simulink model "GNC_exp"  (R2018a)
settings: Solver=FixedStepAuto  StartTime=0.0  StopTime=50  FixedStep=0.05  MaxStep=0.5  MinStep=0.3  RelTol=10  AbsTol=10
values from neighbouring files (symbols this model uses):
  flightplan = [0,2*dist,height,deg2rad(180) ... (first row only)    [initialize_exp.m]    (also in initialize_race_flighttest.m; initialize_race_realtime.m = [dist,0,height,deg2rad(090))
  g = 9.81    [initialize_exp.m]    (also in initialize_race_flighttest.m; initialize_race_realtime.m)
  max_rot_Z = max_vel*(60)*pi/180    (= 0.523598775598)    [initialize_exp.m]    (also in initialize_race_flighttest.m; initialize_race_realtime.m = 1.57079632679)
  max_theta_X = 75*pi/180    (= 1.308996939)    [initialize_exp.m]    (also in initialize_race_flighttest.m; initialize_race_realtime.m)
  max_theta_Y = 75*pi/180    (= 1.308996939)    [initialize_exp.m]    (also in initialize_race_flighttest.m; initialize_race_realtime.m)
  max_v_Z = 2*max_vel    (= 1)    [initialize_exp.m]    (also in initialize_race_flighttest.m; initialize_race_realtime.m = 3)
  max_vel = 0.5    [initialize_exp.m]    (also in initialize_race_flighttest.m; initialize_race_realtime.m = 1.5)
  spline_init = [P0;P1;P2;P3]    [initialize_exp.m]    (also in initialize_race_flighttest.m; initialize_race_realtime.m)
undefined symbols (not defined in the file or in its folder): eul, HFOV, pos, two_std_dev_init, two_std_dev_thres, vel, VFOV, WP_list_init
libraries: sharedtransform x3, aerolibutil x2, simulink x1
(part 2 of 2)

== system GNC_exp/Navigation/calculate desired/calculate direction B'(d)/Make Unit ==
  Vector : Inport
  Multiply : Product
  Reciprocal Sqrt : Sqrt  Operator=rSqrt  SaturateOnIntegerOverflow=on
  Square : Math  Operator=square  SaturateOnIntegerOverflow=on
  Sum of Elements : Sum  Inputs=+
  Transpose : Math  Operator=transpose  SaturateOnIntegerOverflow=on
  Unit Vector : Outport
  wires:
  Reciprocal Sqrt/1 -> Multiply/1
  Vector/1 -> Square/1, Multiply/2
  Square/1 -> Sum of Elements/1
  Multiply/1 -> Transpose/1
  Sum of Elements/1 -> Reciprocal Sqrt/1
  Transpose/1 -> Unit Vector/1

== system GNC_exp/Navigation/calculate desired/calculate direction B'(d)/old, quadratic ==
  note: B'(d) = 2(1-d)(P1-P0) + 2d(P2-P1) = 2*(dP0-2dP1+dP2+P1-P0)
  d : Inport
  P0 : Inport  Port=2
  P1 : Inport  Port=3
  P2 : Inport  Port=4
  vel : Inport  Port=5
  Add1 : Sum  Commented=on  Inputs=+--++-
  Atan1 : Trigonometry  Commented=on  Operator=atan2
  Constant1 : Constant  Commented=on  Value=0
  Constant2 : Constant  Commented=on  Value=0
  Matrix Multiply : Product  Commented=on  Inputs=/*  Multiplication=Matrix(*)
  Product : Product  Commented=on
  Product1 : Product  Commented=on
  Product2 : Product  Commented=on
  Rotation Angles to Direction Cosine Matrix1 : sharedtransform/Rotation Angles to Direction Cosine Matrix  Commented=on  rotationOrder=ZYX  aMode=aMode
      settings: SourceProductBaseCode=AE
  Selector7 : Selector  Commented=on  IndexMode=Zero-based  InputPortWidth=3  IndexOptions=Index vector (dialog)  Indices=1  OutputSizes=1
  Selector8 : Selector  Commented=on  IndexMode=Zero-based  InputPortWidth=3  IndexOptions=Index vector (dialog)  Indices=0  OutputSizes=1
  Vector Concatenate : Concatenate  Commented=on  NumInputs=3
  Vector Concatenate1 : Concatenate  Commented=on  NumInputs=3
  Out1 : Outport
  wires:
  Product2/1 -> Add1/4
  P1/1 -> Add1/5, Product1/2
  Rotation Angles to Direction Cosine Matrix1/1 -> Matrix Multiply/1  "rot matrix"
  P2/1 -> Product2/2
  Add1/1 -> Selector8/1, Selector7/1
  Product/1 -> Add1/1
  P0/1 -> Add1/6, Product/2
  d/1 -> Product2/1, Product1/1, Product/1
  Constant1/1 -> Vector Concatenate/2, Vector Concatenate/3
  Vector Concatenate1/1 -> Matrix Multiply/2
  Product1/1 -> Add1/3, Add1/2
  Vector Concatenate/1 -> Rotation Angles to Direction Cosine Matrix1/1
  Selector7/1 -> Atan1/1
  vel/1 -> Vector Concatenate1/1
  Constant2/1 -> Vector Concatenate1/2, Vector Concatenate1/3
  Matrix Multiply/1 -> Out1/1
  Selector8/1 -> Atan1/2
  Atan1/1 -> Vector Concatenate/1  "yaw"

== system GNC_exp/Navigation/calc v/Create Path Frame/Make X Vector/Make Unit ==
  Vector : Inport
  Multiply : Product
  Reciprocal Sqrt : Sqrt  Operator=rSqrt  SaturateOnIntegerOverflow=on
  Square : Math  Operator=square  SaturateOnIntegerOverflow=on
  Sum of Elements : Sum  Inputs=+
  Unit Vector : Outport
  wires:
  Reciprocal Sqrt/1 -> Multiply/1
  Vector/1 -> Square/1, Multiply/2
  Square/1 -> Sum of Elements/1
  Multiply/1 -> Unit Vector/1
  Sum of Elements/1 -> Reciprocal Sqrt/1

== system GNC_exp/Navigation/calc v/Create Path Frame/Make Y Vector/Make Unit ==
  Vector : Inport
  Multiply : Product
  Reciprocal Sqrt : Sqrt  Operator=rSqrt  SaturateOnIntegerOverflow=on
  Square : Math  Operator=square  SaturateOnIntegerOverflow=on
  Sum of Elements : Sum  Inputs=+
  Unit Vector : Outport
  wires:
  Reciprocal Sqrt/1 -> Multiply/1
  Vector/1 -> Square/1, Multiply/2
  Square/1 -> Sum of Elements/1
  Multiply/1 -> Unit Vector/1
  Sum of Elements/1 -> Reciprocal Sqrt/1

== system GNC_exp/Navigation/calc v/Create Path Frame/Make Z Vector/Make Unit ==
  Vector : Inport
  Multiply : Product
  Reciprocal Sqrt : Sqrt  Operator=rSqrt  SaturateOnIntegerOverflow=on
  Square : Math  Operator=square  SaturateOnIntegerOverflow=on
  Sum of Elements : Sum  Inputs=+
  Unit Vector : Outport
  wires:
  Reciprocal Sqrt/1 -> Multiply/1
  Vector/1 -> Square/1, Multiply/2
  Square/1 -> Sum of Elements/1
  Multiply/1 -> Unit Vector/1
  Sum of Elements/1 -> Reciprocal Sqrt/1

== matlab function GNC_exp/Guidance/filter_WP_moving_av1 ==
  data: WP_list_out output; WP_idx_out output; WP_list_in input; WP_idx_in input; WP_std_dev_in input; dist_old_raw input; WP_current_pos input; WP_current_eul input; WP_std_dev_out output; init_std_dev input; flightplan input
function [WP_list_out, WP_idx_out, WP_std_dev_out] = filter_WP(WP_list_in, WP_idx_in, WP_std_dev_in, dist_old_raw, WP_current_pos, WP_current_eul, init_std_dev, flightplan)
    
%     WP_list_out = zeros(4,4);
%     WP_std_dev_out = zeros(4,1);
   
    % catch state transition
    WP_idx_out = WP_idx_in;
    if dist_old_raw > 1
        disp('new state')
        WP_idx_out = WP_idx_out+1;
        if WP_idx_out == size(WP_list_in,1)
            WP_idx_out = 0;
        end
        WP_std_dev_in = init_std_dev;
    end
    
    WP_std_dev_out = WP_std_dev_in;
    
    % check if there is gate information
    if isequal(WP_current_eul, zeros(1,3)) || isequal(WP_current_eul, zeros(3,1))
        % no gate info
%         disp('gate_global - no corners')
        WP_list_out = WP_list_in;
    else
        % gate info, update WP
%         disp('gate_global - update')
%         WP_current_ori
        lambda = 0.1;
        
        WP_average = WP_list_in(WP_idx_out+1,:)';
        WP_current = [WP_current_pos; WP_current_eul(1)];
       
        delta = WP_current-WP_average;
        delta(4) = angle_add(WP_current(4),-WP_average(4));
        if delta(4) > pi/2
            delta(4) = delta(4)-pi;
        elseif delta(4) < -pi/2
            delta(4) = delta(4)+pi;
        end
        std = abs(delta) ./ (WP_std_dev_out); 
    
        alpha = lambda.^(std);
        alpha = min(alpha, lambda);
%         alpha = max(alpha, 0.001);
        WP_average(1:3) = WP_average(1:3) + alpha(1:3).*delta(1:3);
        WP_average(4) = angle_add(WP_average(4),alpha(4)*delta(4));
        
        WP_std_dev_out = sqrt((1-alpha).*(WP_std_dev_out.^2+alpha.*delta.*delta));

        %WP_list_out(WP_idx_out+1,:) = WP_average;
        
        % update all WP based on new estimate
        WP_list_out = WP_list_in;
        WP_list_out(WP_idx_out+1,:) = WP_average;
        for i = WP_idx_out+2:size(WP_list_in,1)
            WP_list_out(i,1:3) = WP_list_out(i-1,1:3) + flightplan(i,1:3);
            WP_list_out(i,4) = flightplan(i,4);
        end
        if WP_idx_out ~= 0
            WP_list_out(1,1:3) = WP_list_out(end,1:3) + flightplan(1,1:3);
            WP_list_out(1,4) = flightplan(1,4);
            for i = 2:WP_idx_out
                WP_list_out(i,1:3) = WP_list_out(i-1,1:3) + flightplan(i,1:3);
                WP_list_out(i,4) = flightplan(i,4);
            end
        end
        
    end
end

function sum = angle_add(a1,a2)
    sum = atan2(sin(a1+a2),cos(a1+a2));
end



% 
%         if norm(WP_current_pos' - WP_average_pos) < 0.7
%             WP_average_pos = alpha*WP_current_pos' + (1-alpha)*WP_average_pos;
%             WP_current_hdg = WP_current_ori(1);
%             WP_average_hdg = atan2(alpha*sin(WP_current_hdg) + (1-alpha)*sin(WP_average_hdg), ...
%                 alpha*cos(WP_current_hdg) + (1-alpha)*cos(WP_average_hdg));
%             WP_average = [WP_average_pos, WP_average_hdg];
%             WP_list_out(state0_out+1,:) = WP_average;
%         end

== matlab function GNC_exp/Initialize/reset_plot ==
function reset_plot()
coder.extrinsic('quiver3')
coder.extrinsic('legend')
close all;
figure('units','normalized','outerposition',[0 0 0.5 1])
hold on
grid on
axis equal

legends=zeros(12,1);
legends(1)=plot3(0,0,-100,'m.','MarkerSize',7);
legends(2)=plot3(0,0,-100,'k.','MarkerSize',5);
legends(3)=quiver3(0,0,-100,0,0,0,0,'c','MaxHeadSize',1,'LineWidth',2);
legends(4)=quiver3(0,0,-100,0,0,0,0,'r','MaxHeadSize',1,'LineWidth',2);
legends(5)=plot3(0,0,-100,':','Color',[1,0.7,0],'LineWidth',2);
legends(6)=plot3(0,0,-100,'kx-','LineWidth',1.2,'MarkerIndices',1,'MarkerSize',10);
legends(7)=plot3(0,0,-100,'r--','LineWidth',1.5);
legends(8)=plot3(0,0,-100,'g--','LineWidth',1.5);
legends(9)=plot3(0,0,-100,'b--','LineWidth',1.5);
legends(10)=plot3(0,0,-100,'b+-','LineWidth',1.2,'MarkerIndices',1,'MarkerSize',10);
legends(11)=quiver3(0,0,-100,0,0,0,0,'b','MaxHeadSize',1,'LineWidth',2);
legends(12)=plot3(0,0,-100,':r','LineWidth',1);
legend(legends(1:12),'flown track','ground track','inactive WP +ori','active WP +ori','spline','drone pos+vel','drone x','drone y','drone z','des pos+vel','measured WP','std dev (x,y,th)','Location','eastoutside','AutoUpdate','off')

for i=1:25
    plot3(0,0,-100,'.')
end

% axis([-5,5,-5,5,-2,2])
axis([-2,6,-3,1,-1,3])
% axis([1,4,-2,2,0,4])
%view(-20,40) % 3D view
view(-90,90) % top view
%view(-90,0) % front view
xlabel('x')
ylabel('y')
zlabel('z')

== matlab function GNC_exp/Navigation/select d ==
  data: d_old input; d_old output; std_dev input; two_std_dev_thres input
function d_old = select_d(d_old, std_dev, two_std_dev_thres)

two_std_dev_max = 2*max(std_dev.*[1;1;1;1/(40*pi/180)]);

if two_std_dev_max > two_std_dev_thres
    d_old = 0;
end

== matlab function GNC_exp/Plot ==
  data: inbus input
function plot3d(inbus)
%#codegen
coder.extrinsic('delete')
% coder.extrinsic('ellipsoid')
% coder.extrinsic('viscircles')
% coder.extrinsic('quiver3')
% coder.extrinsic('legend')

drone_vel = inbus.state.vel;
drone_pos = inbus.state.pos;
drone_ori = inbus.state.eul;
WP_curr_eul = inbus.WP_curr.eul;
WP_curr_pos = inbus.WP_curr.pos;
SP_des_vel = inbus.SP_des.vel;
SP_des_pos = inbus.SP_des.pos;
WP_idx = inbus.WP_all.idx + 1;
WP_list = inbus.WP_all.list;
effort = inbus.effort;
std_dev = inbus.std_dev;
current_spline = inbus.current_spline;

children = get(gca, 'children');
amount = 12+size(WP_list,1);
delete(children(1:amount));

P0 = current_spline(1,:);
P1 = current_spline(2,:);
P2 = current_spline(3,:);
P3 = current_spline(4,:);

% flown track + ground track
plot3(drone_pos(1),drone_pos(2),drone_pos(3),'m.','MarkerSize',7); %1
% plot3(drone_pos(1),drone_pos(2),0,'k.','MarkerSize',5); %2

% all WPts + ori
% quiver3 (WP_list(:,1),WP_list(:,2),WP_list(:,3),cos(WP_list(:,4)),sin(WP_list(:,4)),zeros(4,1),0,'c','MaxHeadSize',1,'LineWidth',2); %3
for i = 1:size(WP_list,1)
    if i == WP_idx
        continue
    end
    plot3(WP_list(i,1)+[0 cos(WP_list(i,4))],WP_list(i,2)+[0 sin(WP_list(i,4))],WP_list(i,3)+[0 0],'c+-','LineWidth',2,'MarkerIndices',2); %3
end

% WP average pos+ori
% quiver3(P2(1),P2(2),P2(3),cos(P2(4)),sin(P2(4)),0,0,'r','MaxHeadSize',1,'LineWidth',2); %4
plot3(WP_list(WP_idx,1)+[0 cos(WP_list(WP_idx,4))],WP_list(WP_idx,2)+[0 sin(WP_list(WP_idx,4))],WP_list(WP_idx,3)+[0 0],'r+-','LineWidth',2,'MarkerIndices',2); %3

% spline
d = (0:0.05:1)';
% u = ones(1,3);
% spline_pos_quad = (1-d)*u.*((1-d)*P0+d*P1)+d*u.*((1-d)*P1 + d*P2);
spline_pos_cubic = (1-d).^3*P0 + 3*(1-d).^2.*d*P1 + 3*(1-d).*d.^2*P2 + d.^3*P3;
plot3(spline_pos_cubic(:,1),spline_pos_cubic(:,2),spline_pos_cubic(:,3),':','Color',[1,0.7,0],'LineWidth',2); %5
plot3(current_spline(:,1),current_spline(:,2),current_spline(:,3),'og')

% drone pos+vel
plot3(drone_pos(1)+[0 drone_vel(1)],drone_pos(2)+[0 drone_vel(2)],drone_pos(3)+[0 drone_vel(3)],'kx-','LineWidth',1.2,'MarkerIndices',1,'MarkerSize',10); %6

% drone ori
gRb = eul2rotm([drone_ori(3),drone_ori(2),drone_ori(1)]);
length = 1;
x_bebop = gRb*[length;0;0];
y_bebop = gRb*[0;length;0];
z_bebop = gRb*[0;0;length];
plot3(drone_pos(1)+x_bebop(1)*[0.2 1],drone_pos(2)+x_bebop(2)*[0.2 1],drone_pos(3)+x_bebop(3)*[0.2 1],'r:','LineWidth',1.5); %7
plot3(drone_pos(1)+y_bebop(1)*[0.2 1],drone_pos(2)+y_bebop(2)*[0.2 1],drone_pos(3)+y_bebop(3)*[0.2 1],'g:','LineWidth',1.5); %8
plot3(drone_pos(1)+z_bebop(1)*[0.2 1],drone_pos(2)+z_bebop(2)*[0.2 1],drone_pos(3)+z_bebop(3)*[0.2 1],'b:','LineWidth',1.5); %9

% nav pt pos+vel, (yaw)
plot3(SP_des_pos(1)+[0 SP_des_vel(1)],SP_des_pos(2)+[0 SP_des_vel(2)],SP_des_pos(3)+[0 SP_des_vel(3)],'b+-','LineWidth',1.2,'MarkerIndices',1,'MarkerSize',10); %10
% plot3(WP_pos(1)+[0 0.5*cos(WP_yaw)],WP_pos(2)+[0 0.5*sin(WP_yaw)],WP_pos(3)+[0 0],'r-','LineWidth',1)

% WP current pos + ori
if isequal(WP_curr_eul, zeros(1,3)) || isequal(WP_curr_eul, zeros(3,1))
    % no gate info
    WP_curr_pos = [0,0,-100]';
    x_gate = WP_curr_eul;
else   
    gate_rot = eul2rotm(WP_curr_eul');
    x_gate = gate_rot(:,1);
end
% quiver3(gate_pos_global(1),gate_pos_global(2),gate_pos_global(3),x_gate(1),x_gate(2),x_gate(3),0,'b','MaxHeadSize',1,'LineWidth',2); %11
plot3(WP_curr_pos(1)+[0 x_gate(1)],WP_curr_pos(2)+[0 x_gate(2)],WP_curr_pos(3)+[0 x_gate(3)],'b+-','LineWidth',2,'MarkerIndices',2); %3

% effort
effort_gl = ones(4,1) * drone_pos' + [zeros(1,3);
    x_bebop'*effort(1);
    y_bebop'*effort(2);
    z_bebop'*effort(3)];
plot3(effort_gl([1 2],1),effort_gl([1 2],2),effort_gl([1 2],3),'r-','LineWidth',2);
plot3(effort_gl([1 3],1),effort_gl([1 3],2),effort_gl([1 3],3),'g-','LineWidth',2);
plot3(effort_gl([1 4],1),effort_gl([1 4],2),effort_gl([1 4],3),'b-','LineWidth',2);

% WP std dev
two_std_dev = 2*std_dev;
r=linspace(WP_list(WP_idx,4),WP_list(WP_idx,4)+2*pi,4*4*2+1)';
angle_std_dev_length=0.6;
angle_std_dev_draw = [WP_list(WP_idx,1:3);
    WP_list(WP_idx,1:3)+angle_std_dev_length*[cos(WP_list(WP_idx,4)+two_std_dev(4)), sin(WP_list(WP_idx,4)+two_std_dev(4)), 0];
    WP_list(WP_idx,1:3);
    WP_list(WP_idx,1:3)+angle_std_dev_length*[cos(WP_list(WP_idx,4)-two_std_dev(4)), sin(WP_list(WP_idx,4)-two_std_dev(4)), 0];
    WP_list(WP_idx,1:3);
    WP_list(WP_idx,1)+two_std_dev(1)*cos(atan2(two_std_dev(1)/two_std_dev(2)*sin(r),cos(r))), WP_list(WP_idx,2)+two_std_dev(2)*sin(atan2(two_std_dev(1)/two_std_dev(2)*sin(r),cos(r))), WP_list(WP_idx,3)+0*r];
d = angle_std_dev_draw;
plot3(d(:,1),d(:,2),d(:,3),':r','LineWidth',1); %12
% [ellx,elly,ellz] = ellipsoid(P2(1),P2(2),P2(3),3*std_dev(1),3*std_dev(2),3*std_dev(3),20);
% surf(ellx,elly,ellz,ellz,'FaceAlpha',0.5)

% legend
% legend(legends(1:12),'flown track','ground track','inactive WP +ori','active WP +ori','spline','drone pos+vel','drone x','drone y','drone z','des pos+vel','measured WP','std dev (x,y,th)','Location','eastoutside')

== matlab function GNC_exp/Guidance/select_WP ==
  data: WP_average output; WP_list input; WP_idx input
function WP_average = select_WP(WP_list, WP_idx)
    WP_average=zeros(1,4);
    WP_last=zeros(1,4);
    
    WP_average = WP_list(WP_idx+1,:);
    if WP_idx > 0
        WP_last = WP_list(WP_idx,:);
    else
        WP_last = WP_list(end,:);
    end
end

== matlab function GNC_exp/Guidance/create_spline ==
  data: old_spline input; WP_average input; current_spline output size=[4,3]; std_dev input; d_old_raw input; two_std_dev_thres input; VFOV input; HFOV input
function current_spline = create_spline(old_spline, WP_average, std_dev, d_old_raw, two_std_dev_thres, VFOV, HFOV)

two_std_dev_hor = 2*max(std_dev(1:2));
two_std_dev_vert = 2*max(std_dev(3));
two_std_dev_hor = min(2,two_std_dev_hor);
two_std_dev_vert = min(2,two_std_dev_vert);
two_std_dev_max = 2*max(std_dev.*[1;1;1;1/(40*pi/180)]);

% d_old = mod(d_old_raw,1);

SP_pos = (1-d_old_raw)^3*old_spline(1,:) + 3*(1-d_old_raw)^2*d_old_raw*old_spline(2,:) + 3*(1-d_old_raw)*d_old_raw^2*old_spline(3,:) + d_old_raw^3*old_spline(4,:);
SP_vel = 3*(1-d_old_raw)^2*(old_spline(2,:)-old_spline(1,:)) + 6*(1-d_old_raw)*d_old_raw*(old_spline(3,:)-old_spline(2,:)) + 3*d_old_raw^2*(old_spline(4,:)-old_spline(3,:));
SP_vel0= old_spline(2,:)-old_spline(1,:);

WP_gate = WP_average;
offsetH = (two_std_dev_hor+0.7)/sin(HFOV/2);
offsetV = (two_std_dev_vert+0.7)/tan(VFOV/2);
offsetMAX = max(offsetH,offsetV);
if two_std_dev_max > two_std_dev_thres
    WP1 = [SP_pos, atan2(SP_vel(2),SP_vel(1))];
    WP2 = WP_gate(1:4);
    WP2(1:3) = WP_gate(1:3) - offsetMAX*[cos(WP2(4)) sin(WP2(4)) 0];
else
    WP1 = [old_spline(1,:), atan2(SP_vel0(2),SP_vel0(1))];
    WP2 = WP_gate(1:4);
end
    

%% position cubic spline start at supposed pos, random values
% % B(d) = (1-d)^3*P0 + 3(1-d)^2*d*P1 + 3(1-d)*d^2*P2 + d^3*P3
% % B'(d) = 3(1-d)^2(P1-P0) + 6*(1-d)*d*(P2-P1) + 3d^2(P3-P2)
% 
% % B(0) = P0
% % B(1) = P3
% 
% P0 = WP1(1:3);
% P3 = WP2(1:3);
% hdg0 = WP1(4);
% hdg3 = WP2(4);
% 
% m = norm(P0-P3)-1;
% m = max(0.01,m);+
% P1 = [P0(1)+m*cos(hdg0), P0(2)+m*sin(hdg0), P3(3)];
% 
% offset2 = (std_dev_factor+0.7)/sin(HFOV/2*0.999);
% P2 = WP_average(1:3) - (offset2+1*(offset2-offset1))*[cos(hdg3) sin(hdg3) 0];
%           
% % n = 3-norm(P0-WP_average(1:3));
% % n = max(0.001,n);
% % P2 = P3 - n*[cos(WP2(4)) sin(WP2(4)) 0];
% 
% current_spline = [P0; P1; P2; P3];

%% cube with m = n
% % B(d) = (1-d)^3*P0 + 3(1-d)^2*d*P1 + 3(1-d)*d^2*P2 + d^3*P3
% % B'(d) = 3(1-d)^2(P1-P0) + 6*(1-d)*d*(P2-P1) + 3d^2(P3-P2)
% 
% % B(0) = P0
% % B(1) = P3
% 
% P0 = WP1(1:3);
% P3 = WP2(1:3);
% hdg0 = WP1(4);
% hdg3 = WP2(4);
% 
% % g1: P0 + m*[cos(hdg0);sin(hdg0);0]
% % g2: P3 - n*[cos(hdg3);sin(hdg3);0]
% 
% % m*f(hdg0)+n*f(hdg3) +P0-P3 = 0
% % m*(f(hdg0)+f(hdg3)) +P0-P3 = 0
% 
% % m*(c0+c3)+P0(1)-P3(1)=0
% % m = (P3(1)-P0(1) )/(cos(hdg0)+cos(hdg3))
% 
% m = (P3(1)-P0(1) )/(cos(hdg0)+cos(hdg3));
% P1 = P0 + [m*cos(hdg0), m*sin(hdg0), 1*(P3(3)-P0(3))];
% P2 = P3 - [m*cos(hdg3), m*sin(hdg3), 0              ];
% 
% current_spline = [P0; P1; P2; P3];

%% cube without m=n
% % B(d) = (1-d)^3*P0 + 3(1-d)^2*d*P1 + 3(1-d)*d^2*P2 + d^3*P3
% % B'(d) = 3(1-d)^2(P1-P0) + 6*(1-d)*d*(P2-P1) + 3d^2(P3-P2)
% 
% % B(0) = P0
% % B(1) = P3
% 
% P0 = WP1(1:3);
% P3 = WP2(1:3);
% hdg0 = WP1(4);
% hdg3 = WP2(4);
% 
% % g1: P0 + m*[cos(hdg0);sin(hdg0);0]
% % g2: P3 - n*[cos(hdg3);sin(hdg3);0]
% 
% % m*cos(hdg0)+n*cos(hdg3) +P0(1)-P3(1) = 0
% % m*sin(hdg0)+n*sin(hdg3) +P0(2)-P3(2) = 0
% 
% A = [cos(hdg0) cos(hdg3);
%      sin(hdg0) sin(hdg3)];
% b = -[P0(1)-P3(1);
%     P0(2)-P3(2)];
% r = A\b;
% m = r(1);
% n = r(2);
% P1 = P0 + [m*cos(hdg0), m*sin(hdg0), 1*(P3(3)-P0(3))];
% P2 = P3 - [n*cos(hdg3), n*sin(hdg3), 0];
% 
% current_spline = [P0; P1; P2; P3];

%% cube, m and n from dist
% B(d) = (1-d)^3*P0 + 3(1-d)^2*d*P1 + 3(1-d)*d^2*P2 + d^3*P3
% B'(d) = 3(1-d)^2(P1-P0) + 6*(1-d)*d*(P2-P1) + 3d^2(P3-P2)

% B(0) = P0
% B(1) = P3

P0 = WP1(1:3);
P3 = WP2(1:3);
hdg0 = WP1(4);
hdg3 = WP2(4);

% dist_fly = norm(P0-P3);
% dist_nofly = norm(WP_gate(1:3)-P3);
% fact_nofly = max(0.25,sqrt(dist_nofly/2));
% 
% m = dist_fly/4*fact_nofly;
% n = dist_fly/4/fact_nofly;

l_F = norm(P0-P3);
l_TW = norm(WP_gate(1:3)-P3);

m = l_F*min(1/10+l_TW/10,1/2);
n = l_F*max(1-l_TW/2,1/10);

P1 = P0 + [m*cos(hdg0), m*sin(hdg0), 1*(P3(3)-P0(3))];
P2 = P3 - [n*cos(hdg3), n*sin(hdg3), 0];

current_spline = [P0; P1; P2; P3];
end

== matlab function GNC_exp/Guidance/filter_WP_moving_av ==
  data: WP_list_out output; WP_idx_out output; WP_list_in input; WP_idx_in input; dist_old_raw input; WP_current_pos input; WP_current_eul input; WP_std_dev_out output; WP_est_out output; WP_P_mat_out output; two_init_std_dev input; WP_list_const input; WP_est_in input; WP_P_mat_in input
function [WP_list_out, WP_idx_out, WP_std_dev_out, WP_est_out, WP_P_mat_out] = ...
    filter_WP(WP_list_in, WP_idx_in, dist_old_raw, WP_current_pos, WP_current_eul, two_init_std_dev, WP_list_const, WP_est_in, WP_P_mat_in)
    
    mean_var = diag(0.2*ones(4,1));
    
    % catch script start
    if isequal(WP_P_mat_in,ones(4,4))
        WP_P_mat_in = diag((two_init_std_dev/2).^2);
        WP_est_in = WP_list_const(1,:)';
    end
    
    % catch state transition
    WP_idx_out = WP_idx_in;
    if dist_old_raw > 1
        disp('new state')
        WP_idx_out = WP_idx_out+1;
        if WP_idx_out == size(WP_list_in,1)
            WP_idx_out = 0;
        end
        WP_est_in = WP_list_const(WP_idx_out+1,:)';
        %WP_current_gate_in = WP_list_const(WP_idx_out+1,:)';
        WP_P_mat_in = diag((two_init_std_dev/2).^2);
    end
    WP_current_gate = WP_list_const(WP_idx_out+1,:)';
    WP_list_out = WP_list_in;
    
    WP_P_mat_out = WP_P_mat_in;
    WP_std_dev_out = sqrt(diag(WP_P_mat_out));
    
    WP_est_out = WP_est_in;
    
   
    if WP_current_eul(1) > WP_current_gate(4) + pi/2
        euler_used = WP_current_eul(1)-pi;
    elseif WP_current_eul(1) < WP_current_gate(4)-pi/2
        euler_used = WP_current_eul(1)+pi;
    else
        euler_used = WP_current_eul(1);
    end
        
    % check if there is gate information
    if isequal(WP_current_eul, zeros(1,3)) || isequal(WP_current_eul, zeros(3,1))
        % no gate info
        %         disp('gate_global - no corners')
        
    else

        
        if (norm(WP_current_pos(1:2) - WP_current_gate(1:2)) > 2.0) ||...
                WP_current_pos(1) - WP_est_in(1) > 3*sqrt(WP_P_mat_in(1,1)) || ...
                WP_current_pos(2) - WP_est_in(2) > 3*sqrt(WP_P_mat_in(2,2))
                %sqrt(WP_P_mat_in(4,4)) < 0.1 && ...
                %sqrt(WP_P_mat_in(3,3)) < 0.1 && ...
                %sqrt(WP_P_mat_in(2,2)) < 0.1 && ...
                %sqrt(WP_P_mat_in(1,1)) < 0.1) || WP_idx_out ~= WP_idx_out
            %WP_current = [WP_current_pos; WP_current_eul(1)];
            
            %K_gain = WP_P_mat_in*inv(WP_P_mat_in + mean_var);
            
            WP_est_out = WP_est_in;% + K_gain*(WP_current - WP_est_in);
            WP_P_mat_out = WP_P_mat_in;
            
            WP_list_out(WP_idx_out+1,:) = WP_est_out';
            WP_std_dev_out = sqrt(diag(WP_P_mat_out));
            
        else
            
            WP_current = [WP_current_pos; euler_used];
            
            K_gain = WP_P_mat_in*inv(WP_P_mat_in + mean_var);
            
            delta = WP_current-WP_est_in;
            delta(4) = WP_current(4)-WP_est_in(4); %angle_add(WP_current(4),-WP_est_in(4));
            
            WP_est_out(1:3) = WP_est_in(1:3) + K_gain(1:3,:)*(delta);
            WP_est_out(4) = WP_est_in(4) + K_gain(4,:)*delta; %angle_add(WP_est_in(4),K_gain(4,:)*delta);
            WP_P_mat_out = (eye(4) - K_gain)*WP_P_mat_in;
            
            WP_list_out(WP_idx_out+1,:) = WP_est_out';
            WP_std_dev_out = sqrt(diag(WP_P_mat_out));
        end

%         lambda = 0.1;
%         
%         WP_average = WP_list_out(WP_idx_out+1,:)';
%         
%        
%         delta = WP_current-WP_average;
%         delta(4) = angle_add(WP_current(4),-WP_average(4));
%         std = abs(delta) ./ sqrt(WP_std_dev_out);
%     
%         alpha = lambda.^(2*std);
%         alpha = min(alpha, lambda);
% %         alpha = max(alpha, 0.001);
%         WP_average(1:3) = WP_average(1:3) + alpha(1:3).*delta(1:3);
%         WP_average(4) = angle_add(WP_average(4),alpha(4)*delta(4));
%         
%         WP_std_dev_out = sqrt((1-alpha).*(WP_std_dev_out.^2+alpha.*delta.*delta));
% 
%         WP_list_out(WP_idx_out+1,:) = WP_average;
        
    end
end

function sum = angle_add(a1,a2)
    sum = atan2(sin(a1+a2),cos(a1+a2));
end



% 
%         if norm(WP_current_pos' - WP_average_pos) < 0.7
%             WP_average_pos = alpha*WP_current_pos' + (1-alpha)*WP_average_pos;
%             WP_current_hdg = WP_current_ori(1);
%             WP_average_hdg = atan2(alpha*sin(WP_current_hdg) + (1-alpha)*sin(WP_average_hdg), ...
%                 alpha*cos(WP_current_hdg) + (1-alpha)*cos(WP_average_hdg));
%             WP_average = [WP_average_pos, WP_average_hdg];
%             WP_list_out(state0_out+1,:) = WP_average;
%         end

== matlab function GNC_exp/Vision System/gate_global ==
  data: tVec input; rMat input; drone_pos input; drone_ori input; gate_pos_global output; gate_eul_global output
function [gate_pos_global, gate_eul_global]  = gate_global(tVec, rMat, drone_pos, drone_ori)

    gate_pos_global = zeros(3,1);
    gate_eul_global = zeros(3,1);
%     drone_rotm = axang2rotm(drone_ori');
%     gate_pos_local = quatrotate(drone_q,gate_pos_cam);
%     gate_pos_local = drone_rotm * gate_pos_cam';
%     gate_pos_global = gate_pos_local + drone_pos';
%     gate_pos_global = gate_pos_local;

if isequal(tVec,zeros(1,3)) || isequal(tVec,zeros(3,1))
%     disp('gate_global - no corners')
    return
end
    
    %% drone pos
    drone_pos;
    
    %% drone orientation
    dRg = eul2rotm([drone_ori(3),drone_ori(2),drone_ori(1)]);
    
    %% convert gate pos
    % tVec = right down front, drone was front left up
    dRc = eul2rotm([pi/2,-pi/2,0],'ZYX');
    cRd = dRc^-1;
    cRg = dRg*cRd;
    rel= cRg*tVec;
    gate_pos_global = drone_pos + rel;
    
    % rel = -dRs*tvec';
    % gate_pos_global = drone_pos + rel';
    
    %% convert gate orientation
    rot = squeeze(rMat);
    extra = eul2rotm([0,pi/2,0],'ZYX');
    gate_rot = dRg*cRd*rot^-1*extra;
    gate_eul_global = rotm2eul(gate_rot)';
%     
%     wRc = rMat;
%     one_more = 1;%eul2rotm([pi,0,-pi/2]);
%     another_one = 1;%eul2rotm([pi/2,0,0]);
%     wRs = another_one*one_more*cRg*wRc;
%     
%     gate_ori_global = (rotm2eul(wRs))';

%       rot = rMat*cRg^-1;
%       gate_yaw=rotm2eul(rot);
    
end
